simulink model "UpCounter"  (R2025b)
settings: Solver=VariableStepAuto  StartTime=0.0  StopTime=10.0  RelTol=1e-3
settings Model: Creator=Soochan Kim  LastModifiedBy=Soochan Kim

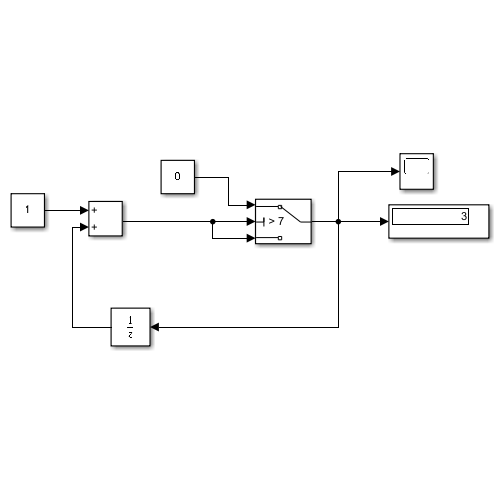
[thumbnail: Simulink's stored preview of the top-level diagram]
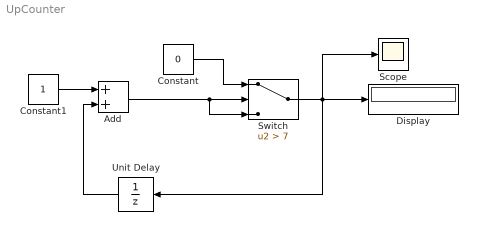
== system UpCounter ==
  Add : Sum
  Constant : Constant  Value=0
  Constant1 : Constant
  Display : Display
  Scope : Scope
      settings: ActiveDisplayYMinimum=-0.87499999999999978  ActiveDisplayYMaximum=7.875
  Switch : Switch  Criteria=u2 > Threshold  Threshold=7  SaturateOnIntegerOverflow=off  InputSameDT=off
  Unit Delay : UnitDelay  SampleTime=-1  HasFrameUpgradeWarning=on
  wires:
  Unit Delay/1 -> Add/2
  Switch/1 -> Unit Delay/1, Scope/1, Display/1
  Add/1 -> Switch/3, Switch/2
  Constant/1 -> Switch/1
  Constant1/1 -> Add/1
